simulink model "inspector"  (R2021b)
settings: Solver=VariableStepAuto  StartTime=0.0  StopTime=inf  RelTol=1e-3
PreLoadFcn:
  | data_inspector_module_setup;
InitFcn:
  | data_inspector_module_setup;
undefined symbols (not defined in the file): AXI4, f_system, Lite
libraries: hdlBasic x25, vmcUtilities x1, simulink x1, dspsigops x1
settings Model: Creator=David Northcote  LastModifiedBy=himan
settings SolverCC: AlgebraicLoopSolver=TrustRegion
settings DebuggingCC: SFMachineParentedDataDiag=warning
settings SFSimCC: CustomCodeUndefinedFunction=UseInterfaceOnly

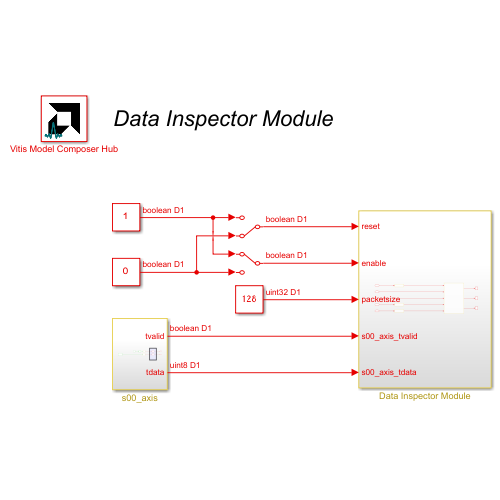
[thumbnail: Simulink's stored preview of the top-level diagram]
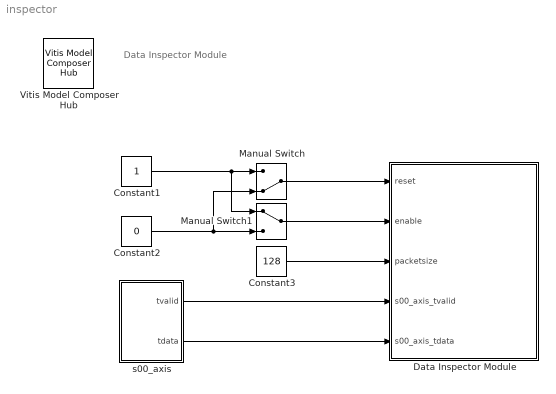
== system inspector ==
  note: Data Inspector Module
  Constant1 : Constant  OutDataTypeStr=boolean  SampleTime=-1
  Constant2 : Constant  Value=0  OutDataTypeStr=boolean  SampleTime=-1
  Constant3 : Constant  Value=128  OutDataTypeStr=uint32  SampleTime=-1
  Data Inspector Module : Subsystem
  Manual Switch : ManualSwitch  CurrentSetting=0
  Manual Switch1 : ManualSwitch
  Vitis Model Composer Hub : vmcUtilities/Vitis Model Composer Hub  Tag=genX  CodeGeneration=off  TargetDirectory=./code  ExportType=System Generator  IpVendor=xilinx.com  IpLibrary=hls  IpVersion=1.0  IpHWLanguage=Verilog  AieCompilerOptions={}  AieSimulatorOptions={}  CreateTestbench=off  TestbenchStackSize=10  RunAieSim=off  AieSimTimeout=50000  RunAieSimProfiling=off  LaunchVitisAnalyzer=off  PlotOutput=off  RunX86Sim=off  X86SimTimeout=10  GenHwImage=off  PlatformType=Not Specified  HwSystemType=Baremetal  HwValidationTarget=hw  ProjDevice=xczu28dr-ffvg1517-2-e  ProjDevicePart=xczu28dr-ffvg1517-2-e  SamplePeriod=-1  ClockFrequency=200  DataPathParallelism=1  xilinxfamily=zynquplusRFSOC  part=xczu28dr  speed=-2-e  package=ffvg1517  directory=./netlist  testbench=off  incr_netlist=off  synthesis_tool=Vivado  clock_wrapper=Clock Enables  dbl_ovrd=According to Block Masks  dcm_input_clock_period=10  sysclk_period=(1/f_system)*1e9  simulink_period=1/f_system  eval_field=0  IPInfoJsonString="{\"HDLSubsystem\":{\"SubsystemName\":\"inspector\",\"IPName\":\"data_inspector_module\",\"IPLibrary\":\"RFSoC\",\"IPVendor\":\"UoS\",\"IPVersion\":\"1.0\"}}"  LogFileName=''  NThreads=4
  s00_axis : Subsystem
  wires:
  Constant1/1 -> Manual Switch1/1, Manual Switch/1
  Constant2/1 -> Manual Switch/2, Manual Switch1/2
  Constant3/1 -> Data Inspector Module/3(packetsize)
  Manual Switch/1 -> Data Inspector Module/1(reset)
  s00_axis/1(tvalid) -> Data Inspector Module/4(s00_axis_tvalid)
  s00_axis/2(tdata) -> Data Inspector Module/5(s00_axis_tdata)
  Manual Switch1/1 -> Data Inspector Module/2(enable)

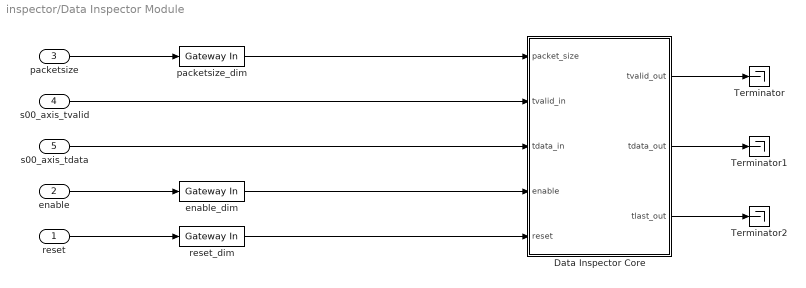
== system inspector/Data Inspector Module ==
  reset : Inport
  enable : Inport  Port=2
  packetsize : Inport  Port=3
  s00_axis_tvalid : Inport  Port=4
  s00_axis_tdata : Inport  Port=5
  Data Inspector Core : Subsystem
  Terminator : Terminator
  Terminator1 : Terminator
  Terminator2 : Terminator
  enable_dim : hdlBasic/Gateway In  gui_display_data_type=Boolean  arith_type=Boolean  n_bits=32  bin_pt=0  preci_type=Single  exp_width=8  frac_width=24  rows=1  columns=1  quantization="Round  (unbiased: +/- Inf)"  overflow=Saturate  period=1/f_system  UseAsADC=off  ADCChannel='1'  interface=AXI4-Lite  automatic_assignment=off  address_offset=4  intf_name=''  intf_description=''  default_value=0  timing_constraint=None  locs_specified=off  LOCs={}  io_standard={}  inherit_from_input=off  hdl_port=on  XmcBlockStatus=1  maskContainerNames=group4  block_type=gatewayin  block_config=sysgen:gateway_in_config  block_width_w=590  block_height_w=620  block_width=640  block_height=850
  packetsize_dim : hdlBasic/Gateway In  gui_display_data_type=Fixed-point  arith_type=Unsigned  n_bits=32  bin_pt=0  preci_type=Single  exp_width=8  frac_width=24  rows=1  columns=1  quantization="Round  (unbiased: +/- Inf)"  overflow=Saturate  period=1/f_system  UseAsADC=off  ADCChannel='1'  interface=AXI4-Lite  automatic_assignment=off  address_offset=8  intf_name=''  intf_description=''  default_value=0  timing_constraint=None  locs_specified=off  LOCs={}  io_standard={}  inherit_from_input=off  hdl_port=on  XmcBlockStatus=1  maskContainerNames=group4  block_type=gatewayin  block_config=sysgen:gateway_in_config  block_width_w=590  block_height_w=620  block_width=640  block_height=850
  reset_dim : hdlBasic/Gateway In  gui_display_data_type=Boolean  arith_type=Boolean  n_bits=16  bin_pt=14  preci_type=Single  exp_width=8  frac_width=24  rows=1  columns=1  quantization="Round  (unbiased: +/- Inf)"  overflow=Saturate  period=1/f_system  UseAsADC=off  ADCChannel='1'  interface=AXI4-Lite  automatic_assignment=off  address_offset=0  intf_name=''  intf_description=''  default_value=0  timing_constraint=None  locs_specified=off  LOCs={}  io_standard={}  inherit_from_input=off  hdl_port=on  XmcBlockStatus=1  maskContainerNames=group4  block_type=gatewayin  block_config=sysgen:gateway_in_config  block_width_w=590  block_height_w=620  block_width=640  block_height=850
  wires:
  Data Inspector Core/2(tdata_out) -> Terminator1/1
  Data Inspector Core/3(tlast_out) -> Terminator2/1
  reset_dim/1 -> Data Inspector Core/5(reset)
  Data Inspector Core/1(tvalid_out) -> Terminator/1
  reset/1 -> reset_dim/1
  packetsize/1 -> packetsize_dim/1
  s00_axis_tdata/1 -> Data Inspector Core/3(tdata_in)
  packetsize_dim/1 -> Data Inspector Core/1(packet_size)
  s00_axis_tvalid/1 -> Data Inspector Core/2(tvalid_in)
  enable_dim/1 -> Data Inspector Core/4(enable)
  enable/1 -> enable_dim/1

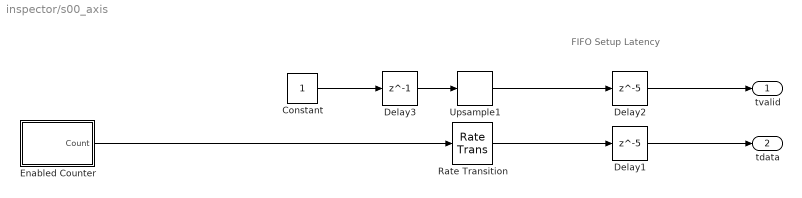
== system inspector/s00_axis ==
  note: FIFO Setup Latency
  Constant : Constant  OutDataTypeStr=boolean  SampleTime=-1
  Delay1 : Delay  DelayLength=5
  Delay2 : Delay  DelayLength=5
  Delay3 : Delay  DelayLength=1
  Enabled Counter : Subsystem  TreatAsAtomicUnit=on
  Rate Transition : RateTransition  OutPortSampleTime=1/f_system
  Upsample1 : dspsigops/Upsample  N=f_system/(400e3)  phase=0  RateOptions=Allow multirate processing  ic=0  mode=Unused parameter value
  tvalid : Outport  VectorParamsAs1DForOutWhenUnconnected=off
  tdata : Outport  Port=2  VectorParamsAs1DForOutWhenUnconnected=off
  wires:
  Delay2/1 -> tvalid/1
  Delay1/1 -> tdata/1
  Enabled Counter/1(Count) -> Rate Transition/1
  Constant/1 -> Delay3/1
  Rate Transition/1 -> Delay1/1
  Upsample1/1 -> Delay2/1
  Delay3/1 -> Upsample1/1

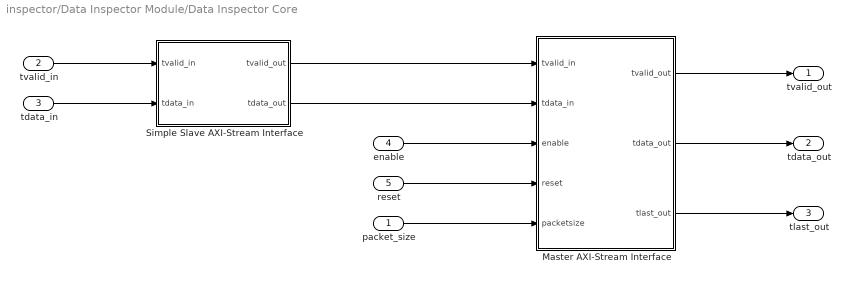
== system inspector/Data Inspector Module/Data Inspector Core ==
  packet_size : Inport
  tvalid_in : Inport  Port=2
  tdata_in : Inport  Port=3
  enable : Inport  Port=4
  reset : Inport  Port=5
  Master AXI-Stream Interface : Subsystem
  Simple Slave AXI-Stream Interface : Subsystem
  tvalid_out : Outport  VectorParamsAs1DForOutWhenUnconnected=off
  tdata_out : Outport  Port=2  VectorParamsAs1DForOutWhenUnconnected=off
  tlast_out : Outport  Port=3  VectorParamsAs1DForOutWhenUnconnected=off
  wires:
  Master AXI-Stream Interface/2(tdata_out) -> tdata_out/1
  Master AXI-Stream Interface/3(tlast_out) -> tlast_out/1
  Master AXI-Stream Interface/1(tvalid_out) -> tvalid_out/1
  tvalid_in/1 -> Simple Slave AXI-Stream Interface/1(tvalid_in)
  tdata_in/1 -> Simple Slave AXI-Stream Interface/2(tdata_in)
  enable/1 -> Master AXI-Stream Interface/3(enable)
  packet_size/1 -> Master AXI-Stream Interface/5(packetsize)
  Simple Slave AXI-Stream Interface/1(tvalid_out) -> Master AXI-Stream Interface/1(tvalid_in)
  Simple Slave AXI-Stream Interface/2(tdata_out) -> Master AXI-Stream Interface/2(tdata_in)
  reset/1 -> Master AXI-Stream Interface/4(reset)

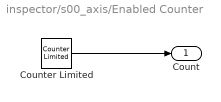
== system inspector/s00_axis/Enabled Counter ==
  Counter Limited : simulink/Sources/Counter Limited  uplimit=127  tsamp=1/(400e3)
  Count : Outport  VectorParamsAs1DForOutWhenUnconnected=off
  wires:
  Counter Limited/1 -> Count/1

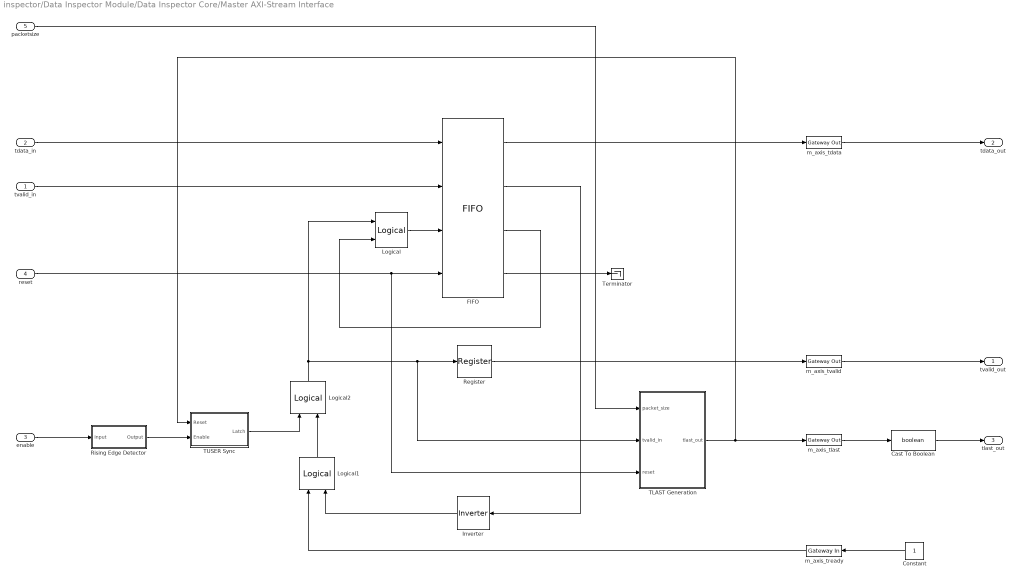
== system inspector/Data Inspector Module/Data Inspector Core/Master AXI-Stream Interface ==
  tvalid_in : Inport
  tdata_in : Inport  Port=2
  enable : Inport  Port=3
  reset : Inport  Port=4
  packetsize : Inport  Port=5
  Cast To Boolean : DataTypeConversion  OutDataTypeStr=boolean
  Constant : Constant  OutDataTypeStr=boolean  SampleTime=1/f_system
  FIFO : hdlBasic/FIFO  mem_type=Block RAM  performance_options=Standard_FIFO  embedded_registers=off  depth=1K  use_asym_data_widths=off  asym_read_width=32  percent_nbits=1  rst=on  rst_latency=2  en=off  use_dcount=on  use_percent_full_port=off  use_almost_empty=off  almost_empty_thresh=2  use_almost_full=off  use_rd_rst_busy=off  use_wr_rst_busy=off  almost_full_thresh=14  almost_empty_offset=[]  almost_full_offset=[]  explicit_period=off  period=[]  store_only_valid=[]  init_zero=[]  simulation_type=fast_sim  XmcBlockStatus=1  maskContainerNames=tabcontainer1  block_type=fifo  block_config=sysgen:FIFO_config  block_width=538  block_height=997
      settings: infoedit=[]
  Inverter : hdlBasic/Inverter  en=off  latency=0  XmcBlockStatus=1  maskContainerNames=group2  block_type=inv  block_config=sysgen:Inverter_config
  Logical : hdlBasic/Logical  logical_function=OR  inputs=2  en=off  latency=0  precision=Full  arith_type=Unsigned  n_bits=16  bin_pt=0  align_bp=on  overflow=[]  quantization=[]  XmcBlockStatus=1  maskContainerNames=tabcontainer1  block_type=logical  block_config=sysgen:Logical_config
  Logical1 : hdlBasic/Logical  logical_function=AND  inputs=2  en=off  latency=0  precision=Full  arith_type=Unsigned  n_bits=16  bin_pt=0  align_bp=on  overflow=[]  quantization=[]  XmcBlockStatus=1  maskContainerNames=tabcontainer1  block_type=logical  block_config=sysgen:Logical_config
  Logical2 : hdlBasic/Logical  logical_function=AND  inputs=2  en=off  latency=0  precision=Full  arith_type=Unsigned  n_bits=16  bin_pt=0  align_bp=on  overflow=[]  quantization=[]  XmcBlockStatus=1  maskContainerNames=tabcontainer1  block_type=logical  block_config=sysgen:Logical_config
  Register : hdlBasic/Register  init=0  rst=off  en=off  XmcBlockStatus=1  maskContainerNames=tabcontainer1  block_type=register  block_config=sysgen:Register_config
  Rising Edge Detector : Subsystem
  TLAST Generation : Subsystem
  TUSER Sync : Subsystem
  Terminator : Terminator
  m_axis_tdata : hdlBasic/Gateway Out  inherit_from_input=on  hdl_port=on  rows=1  columns=1  UseAsDAC=off  DACChannel='1'  interface=None  automatic_assignment=on  address_offset=hex2dec('00')  intf_name=''  intf_description=''  timing_constraint=None  locs_specified=off  LOCs={}  io_standard={}  XmcBlockStatus=1  maskContainerNames=group4  block_type=gatewayout  block_config=sysgen:gateway_out_config  block_width_w=590  block_height_w=620  block_width=620  block_height=750
  m_axis_tlast : hdlBasic/Gateway Out  inherit_from_input=on  hdl_port=on  rows=1  columns=1  UseAsDAC=off  DACChannel='1'  interface=None  automatic_assignment=on  address_offset=hex2dec('00')  intf_name=''  intf_description=''  timing_constraint=None  locs_specified=off  LOCs={}  io_standard={}  XmcBlockStatus=1  maskContainerNames=group4  block_type=gatewayout  block_config=sysgen:gateway_out_config  block_width_w=590  block_height_w=620  block_width=620  block_height=750
  m_axis_tready : hdlBasic/Gateway In  gui_display_data_type=Boolean  arith_type=Boolean  n_bits=16  bin_pt=14  preci_type=Single  exp_width=8  frac_width=24  rows=1  columns=1  quantization="Round  (unbiased: +/- Inf)"  overflow=Saturate  period=1/f_system  UseAsADC=off  ADCChannel='1'  interface=None  automatic_assignment=on  address_offset=hex2dec('00')  intf_name=''  intf_description=''  default_value=0  timing_constraint=None  locs_specified=off  LOCs={}  io_standard={}  inherit_from_input=off  hdl_port=on  XmcBlockStatus=1  maskContainerNames=group4  block_type=gatewayin  block_config=sysgen:gateway_in_config  block_width_w=590  block_height_w=620  block_width=640  block_height=850
  m_axis_tvalid : hdlBasic/Gateway Out  inherit_from_input=on  hdl_port=on  rows=1  columns=1  UseAsDAC=off  DACChannel='1'  interface=None  automatic_assignment=on  address_offset=hex2dec('00')  intf_name=''  intf_description=''  timing_constraint=None  locs_specified=off  LOCs={}  io_standard={}  XmcBlockStatus=1  maskContainerNames=group4  block_type=gatewayout  block_config=sysgen:gateway_out_config  block_width_w=590  block_height_w=620  block_width=620  block_height=750
  tvalid_out : Outport  VectorParamsAs1DForOutWhenUnconnected=off
  tdata_out : Outport  Port=2  VectorParamsAs1DForOutWhenUnconnected=off
  tlast_out : Outport  Port=3  VectorParamsAs1DForOutWhenUnconnected=off
  wires:
  Constant/1 -> m_axis_tready/1
  m_axis_tdata/1 -> tdata_out/1
  m_axis_tvalid/1 -> tvalid_out/1
  m_axis_tlast/1 -> Cast To Boolean/1
  tvalid_in/1 -> FIFO/2
  reset/1 -> TLAST Generation/3(reset), FIFO/4
  Cast To Boolean/1 -> tlast_out/1
  tdata_in/1 -> FIFO/1
  FIFO/2 -> Inverter/1
  Logical/1 -> FIFO/3
  Inverter/1 -> Logical1/2
  FIFO/3 -> Logical/2
  FIFO/4 -> Terminator/1
  m_axis_tready/1 -> Logical1/1
  FIFO/1 -> m_axis_tdata/1
  TLAST Generation/1(tlast_out) -> TUSER Sync/1(Reset), m_axis_tlast/1
  TUSER Sync/1(Latch) -> Logical2/1
  Logical2/1 -> Logical/1, TLAST Generation/2(tvalid_in), Register/1
  Logical1/1 -> Logical2/2
  Rising Edge Detector/1(Output) -> TUSER Sync/2(Enable)
  enable/1 -> Rising Edge Detector/1(Input)
  packetsize/1 -> TLAST Generation/1(packet_size)
  Register/1 -> m_axis_tvalid/1

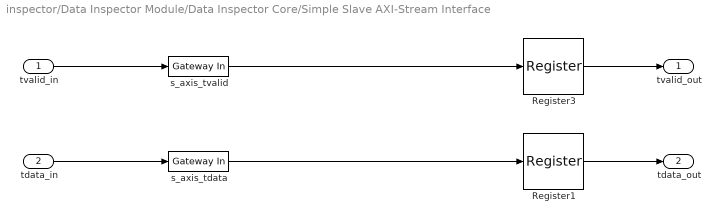
== system inspector/Data Inspector Module/Data Inspector Core/Simple Slave AXI-Stream Interface ==
  tvalid_in : Inport
  tdata_in : Inport  Port=2
  Register1 : hdlBasic/Register  init=0  rst=off  en=off  XmcBlockStatus=1  maskContainerNames=tabcontainer1  block_type=register  block_config=sysgen:Register_config
  Register3 : hdlBasic/Register  init=0  rst=off  en=off  XmcBlockStatus=1  maskContainerNames=tabcontainer1  block_type=register  block_config=sysgen:Register_config
  s_axis_tdata : hdlBasic/Gateway In  gui_display_data_type=Fixed-point  arith_type=Unsigned  n_bits=32  bin_pt=0  preci_type=Single  exp_width=8  frac_width=24  rows=1  columns=1  quantization="Round  (unbiased: +/- Inf)"  overflow=Saturate  period=1/f_system  UseAsADC=off  ADCChannel='1'  interface=None  automatic_assignment=on  address_offset=hex2dec('00')  intf_name=''  intf_description=''  default_value=0  timing_constraint=None  locs_specified=off  LOCs={}  io_standard={}  inherit_from_input=off  hdl_port=on  XmcBlockStatus=1  maskContainerNames=group4  block_type=gatewayin  block_config=sysgen:gateway_in_config  block_width_w=590  block_height_w=620  block_width=640  block_height=850
  s_axis_tvalid : hdlBasic/Gateway In  gui_display_data_type=Boolean  arith_type=Boolean  n_bits=16  bin_pt=14  preci_type=Single  exp_width=8  frac_width=24  rows=1  columns=1  quantization="Round  (unbiased: +/- Inf)"  overflow=Saturate  period=1/f_system  UseAsADC=off  ADCChannel='1'  interface=None  automatic_assignment=on  address_offset=hex2dec('00')  intf_name=''  intf_description=''  default_value=0  timing_constraint=None  locs_specified=off  LOCs={}  io_standard={}  inherit_from_input=off  hdl_port=on  XmcBlockStatus=1  maskContainerNames=group4  block_type=gatewayin  block_config=sysgen:gateway_in_config  block_width_w=590  block_height_w=620  block_width=640  block_height=850
  tvalid_out : Outport  VectorParamsAs1DForOutWhenUnconnected=off
  tdata_out : Outport  Port=2  VectorParamsAs1DForOutWhenUnconnected=off
  wires:
  tdata_in/1 -> s_axis_tdata/1
  s_axis_tdata/1 -> Register1/1
  s_axis_tvalid/1 -> Register3/1
  tvalid_in/1 -> s_axis_tvalid/1
  Register3/1 -> tvalid_out/1
  Register1/1 -> tdata_out/1

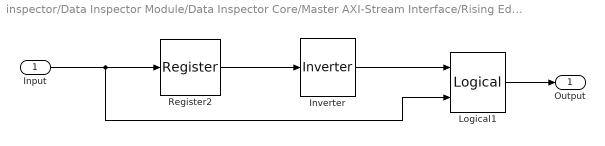
== system inspector/Data Inspector Module/Data Inspector Core/Master AXI-Stream Interface/Rising Edge Detector ==
  Input : Inport
  Inverter : hdlBasic/Inverter  en=off  latency=0  XmcBlockStatus=1  maskContainerNames=group2  block_type=inv  block_config=sysgen:Inverter_config
  Logical1 : hdlBasic/Logical  logical_function=AND  inputs=2  en=off  latency=0  precision=User Defined  arith_type=Boolean  n_bits=16  bin_pt=0  align_bp=on  overflow=[]  quantization=[]  XmcBlockStatus=1  maskContainerNames=tabcontainer1  block_type=logical  block_config=sysgen:Logical_config
  Register2 : hdlBasic/Register  init=0  rst=off  en=off  XmcBlockStatus=1  maskContainerNames=tabcontainer1  block_type=register  block_config=sysgen:Register_config
  Output : Outport  VectorParamsAs1DForOutWhenUnconnected=off
  wires:
  Register2/1 -> Inverter/1
  Inverter/1 -> Logical1/1
  Logical1/1 -> Output/1
  Input/1 -> Logical1/2, Register2/1

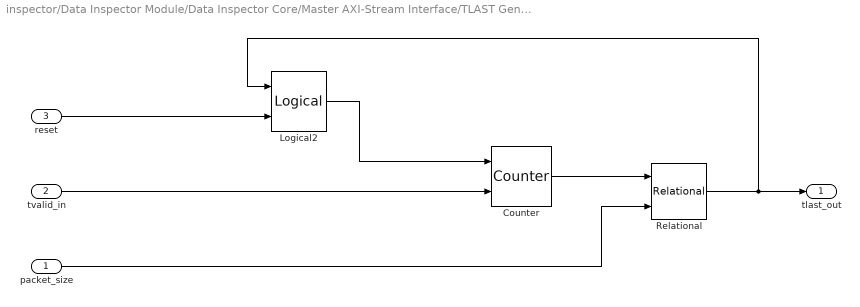
== system inspector/Data Inspector Module/Data Inspector Core/Master AXI-Stream Interface/TLAST Generation ==
  packet_size : Inport
  tvalid_in : Inport  Port=2
  reset : Inport  Port=3
  Counter : hdlBasic/Counter  cnt_type=Free running  cnt_to=Inf  operation=Up  start_count=0  cnt_by_val=1  arith_type=Unsigned  n_bits=32  bin_pt=0  load_pin=off  rst=on  en=on  explicit_period=Inferred from inputs  period=1  use_behavioral_HDL=off  implementation=Fabric  XmcBlockStatus=1  maskContainerNames=group1  block_type=counter  block_config=sysgen:Counter_config  block_width=531  block_height=1023
  Logical2 : hdlBasic/Logical  logical_function=OR  inputs=2  en=off  latency=0  precision=Full  arith_type=Unsigned  n_bits=16  bin_pt=0  align_bp=on  overflow=[]  quantization=[]  XmcBlockStatus=1  maskContainerNames=tabcontainer1  block_type=logical  block_config=sysgen:Logical_config
  Relational : hdlBasic/Relational  mode=a>=b  op_type=Bool  en=off  latency=0  XmcBlockStatus=1  maskContainerNames=tabcontainer1  block_type=relational  block_config=sysgen:Relational_config
  tlast_out : Outport  VectorParamsAs1DForOutWhenUnconnected=off
  wires:
  tvalid_in/1 -> Counter/2
  Logical2/1 -> Counter/1
  reset/1 -> Logical2/2
  Counter/1 -> Relational/1
  packet_size/1 -> Relational/2
  Relational/1 -> tlast_out/1, Logical2/1

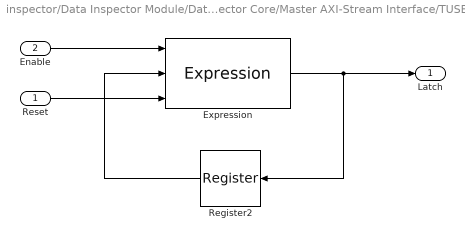
== system inspector/Data Inspector Module/Data Inspector Core/Master AXI-Stream Interface/TUSER Sync ==
  Reset : Inport
  Enable : Inport  Port=2
  Expression : hdlBasic/Expression  expression=(~R)&((Q^E)|(Q&E))  align_bp=on  en=off  latency=0  precision=Full  arith_type=Unsigned  n_bits=16  bin_pt=0  XmcBlockStatus=1  maskContainerNames=tabcontainer1  block_type=expr  block_config=sysgen:Expr_config
  Register2 : hdlBasic/Register  init=0  rst=off  en=off  XmcBlockStatus=1  maskContainerNames=tabcontainer1  block_type=register  block_config=sysgen:Register_config
  Latch : Outport  VectorParamsAs1DForOutWhenUnconnected=off
  wires:
  Register2/1 -> Expression/2
  Expression/1 -> Latch/1, Register2/1
  Enable/1 -> Expression/1
  Reset/1 -> Expression/3
